simulink model "Simulation_main"  (R2018a)
settings: Solver=VariableStepDiscrete  StartTime=0.0  StopTime=0.1  RelTol=1e-3
libraries: powerlib x21, powerlib_meascontrol x1
settings Model: Creator=chama  LastModifiedBy=LENOVO

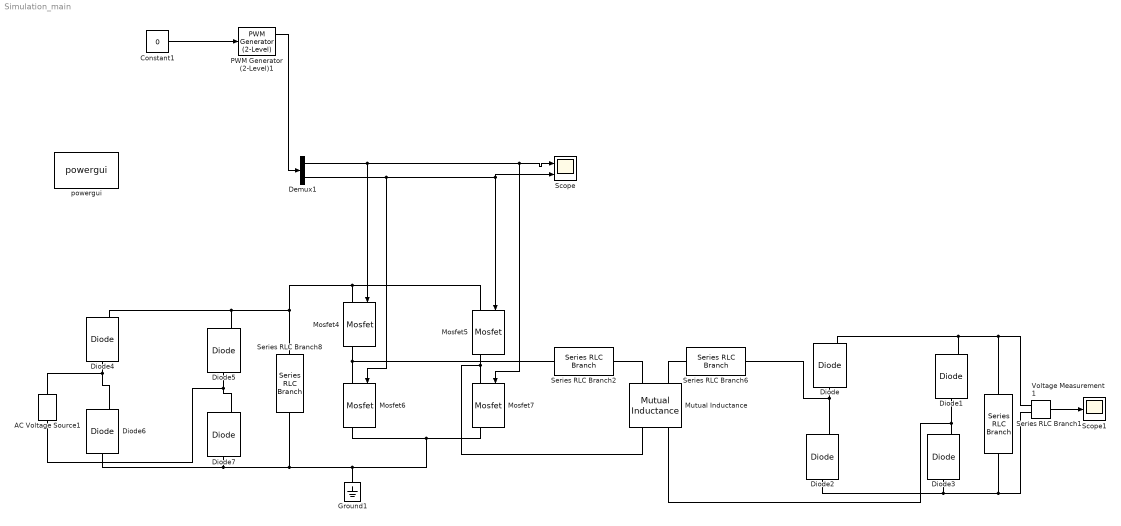
== system Simulation_main ==
  AC Voltage Source1 : powerlib/Electrical Sources/AC Voltage Source  Amplitude=230  Phase=0  Frequency=50  SampleTime=1e-7  Measurements=None  BusType=swing  Pref=10e3  Qref=0  Qmin=-inf  Qmax=+inf
  Constant1 : Constant  Value=0
  Demux1 : Demux  Outputs=2
  Diode{,1..7} (8 alike) : powerlib/Power Electronics/Diode  Ron=0.001  Lon=0  Vf=0.8  IC=0  UseSnubber=0  Rs=500  Cs=250e-9  Measurements=on
  Ground1 : powerlib/Elements/Ground  LConnTagsString=a
  Mosfet{4..7} (4 alike) : powerlib/Power Electronics/Mosfet  Ron=0.1  Lon=0  Rd=0.01  Vfd=0  IC=0  Rs=1e5  Cs=inf  Measurements=on
  Mutual Inductance : powerlib/Elements/Mutual Inductance  LConnTagsString=a|b  RConnTagsString=A|B  TypeOfMutual=Two or three windings with equal mutual terms  NumberOfWindings=3  SelfImpedance1=[1.0 1e-06]  SelfImpedance2=[ 1.0 1e-06]  ThreeWindings=off  SelfImpedance3=[ 1.1 1.1e-03]  MutualImpedance=[0.5 5e-07]  InductanceMatrix="[1.0 0.9  0.9 ;  0.9 1.0  0.9;  0.9 0.9 1.0 ] * 1e-3"  ResistanceMatrix="[1.0 0.9  0.9 ;  0.9 1.0  0.9;  0.9 0.9 1.0 ]"  Measurements=Winding voltages and currents
      settings: AttributesFormatString=\n  SourceProductName=Simscape Power Systems  SourceProductBaseCode=PS
  PWM Generator (2-Level)1 : powerlib_meascontrol/Pulse & Signal Generators/PWM Generator (2-Level)  ModulatorType=Single-phase half-bridge (2 pulses)  ModulatorMode=Unsynchronized  Fc=85e3  Pc=0  nF=27  MinMax="[ -120  120 ]"  SamplingTechnique=Symmetrical regular (single edge)  ModulatingSignals=off  m=0.8  Freq=60  Phase=0  Ts=0  ShowCarrierOutport=on
      settings: SourceProductName=Simscape Power Systems
  Scope : Scope  NumInputPorts=2
  Scope1 : Scope
  Series RLC Branch1 : powerlib/Elements/Series RLC Branch  LConnTagsString=__new0  RConnTagsString=__new0  BranchType=C  Resistance=1  Inductance=1e-3  SetiL0=off  InitialCurrent=0  Capacitance=1e-6  Setx0=off  InitialVoltage=0  Measurements=None
  Series RLC Branch2 : powerlib/Elements/Series RLC Branch  LConnTagsString=__new0  RConnTagsString=__new0  BranchType=C  Resistance=1  Inductance=1e-3  SetiL0=off  InitialCurrent=0  Capacitance=3.5e-6  Setx0=off  InitialVoltage=0  Measurements=None
  Series RLC Branch6 : powerlib/Elements/Series RLC Branch  LConnTagsString=__new0  RConnTagsString=__new0  BranchType=C  Resistance=1  Inductance=1e-3  SetiL0=off  InitialCurrent=0  Capacitance=3.5e-6  Setx0=off  InitialVoltage=0  Measurements=None
  Series RLC Branch8 : powerlib/Elements/Series RLC Branch  LConnTagsString=__new0  RConnTagsString=__new0  BranchType=C  Resistance=1  Inductance=1e-3  SetiL0=off  InitialCurrent=0  Capacitance=1000e-6  Setx0=off  InitialVoltage=0  Measurements=None
  Voltage Measurement1 : powerlib/Measurements/Voltage Measurement  PhasorSimulation=off  OutputType=Complex  PSBequivalent=0
  powergui : powerlib/powergui  Priority=1  SimulationMode=Discrete  SampleTime=1e-7  frequency=60  Iterations=50  frequencyindice=0  Pbase=100e6  ErrMax=1e-4  UnitsV=kV  UnitsW=MW  buscounter=0  FunctionMessages=off  echomessages=off  EnableUseOfTLC=off  CurrentSourceSwitches=off  DisableSnubberDevices=off  DisableRonSwitches=off  DisableVfSwitches=off  DisplayEquations=off  SolverType=Tustin/Backward Euler (TBE)  Interpol=off  ExternalGateDelay=off  methode=off  Ts=100  x0status=blocks  SPID=on  SwTol=0  HookPort=off  RestoreLinks=warning  ResistiveCurrentMeasurement=off  Frange=[0:2:500]  Ylog=off  Xlog=on  ShowGrid=off  save=off  variable=ZData  structure=0  ZoomFFT=off  StartTime=0.0  cycles=1  DisplayStyle=1  fundamental=60  FreqAxis=off  MaxFrequency=1000  frequencyindicesteady=1  RmsSteady=1  display=off
  wires:
  Demux1/2 -> Mosfet6/1, Scope/2, Mosfet5/1
  Constant1/1 -> PWM Generator (2-Level)1/1
  Demux1/1 -> Scope/1, Mosfet7/1, Mosfet4/1
  PWM Generator (2-Level)1/1 -> Demux1/1
  Voltage Measurement1/1 -> Scope1/1
  connections:
  Mosfet7/LConn1 -- Mutual Inductance/RConn1 -- Mosfet5/RConn1
  Mosfet6/LConn1 -- Series RLC Branch2/LConn1 -- Mosfet4/RConn1
  Diode6/LConn1 -- Series RLC Branch8/RConn1 -- Ground1/LConn1 -- Mosfet6/RConn1 -- Mosfet7/RConn1 -- Diode7/LConn1
  Series RLC Branch2/RConn1 -- Mutual Inductance/LConn1
  Series RLC Branch6/LConn1 -- Mutual Inductance/LConn2
  Diode3/RConn1 -- Diode1/LConn1 -- Mutual Inductance/RConn2
  Diode2/RConn1 -- Series RLC Branch6/RConn1 -- Diode/LConn1
  Diode2/LConn1 -- Voltage Measurement1/LConn2 -- Series RLC Branch1/RConn1 -- Diode3/LConn1
  Diode1/RConn1 -- Voltage Measurement1/LConn1 -- Series RLC Branch1/LConn1 -- Diode/RConn1
  Diode7/RConn1 -- AC Voltage Source1/LConn1 -- Diode5/LConn1
  Diode6/RConn1 -- AC Voltage Source1/RConn1 -- Diode4/LConn1
  Series RLC Branch8/LConn1 -- Diode5/RConn1 -- Diode4/RConn1 -- Mosfet4/LConn1 -- Mosfet5/LConn1
